simulink model "Pend_Model"  (Simulink 8.1)
settings: Solver=ode45  StartTime=0.0  StopTime=10.0  RelTol=1e-3
values from neighbouring files (symbols this model uses):
  b = 0.1    [pendulum.m]    (also in pid.m; pid_control.m)
  g = 9.8    [FastAHCCartPole.m]    (also in pendulum.m; pid.m; pid_control.m)
  l = 0.3    [pendulum.m]    (also in pid.m; pid_control.m)
  m = 0.2    [pendulum.m]    (also in pid.m; pid_control.m)
  M = 0.5    [pendulum.m]    (also in pid.m; pid_control.m)
  T = feedback(P_pend,C)    [pendulum.m]    (also in pid.m; pid_control.m)
settings Model: Creator=david78k  LastModifiedBy=david78k
settings DataIOCC: SignalLoggingSaveFormat=Dataset
settings OptimizationCC: ExpressionDepthLimit=128
settings DebuggingCC: FcnCallInpInsideContextMsg=EnableAllAsError
settings GRTTargetCC: CombineOutputUpdateFcns=on  GRTInterface=off

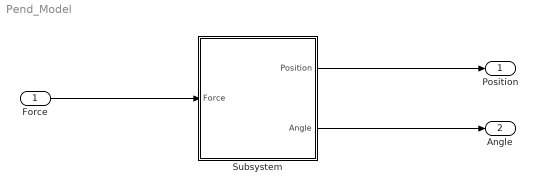
== system Pend_Model ==
  Force : Inport
  Subsystem : Subsystem
  Position : Outport
  Angle : Outport  Port=2
  wires:
  Force/1 -> Subsystem/1(Force)
  Subsystem/1(Position) -> Position/1
  Subsystem/2(Angle) -> Angle/1

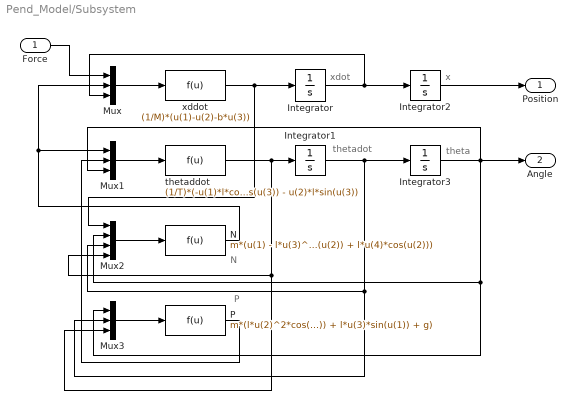
== system Pend_Model/Subsystem ==
  note: P
  note: N
  note: theta
  note: x
  note: thetadot
  note: xdot
  Force : Inport
  Integrator : Integrator  ContinuousStateAttributes='xdot'
  Integrator1 : Integrator  ContinuousStateAttributes='thetadot'
  Integrator2 : Integrator  ContinuousStateAttributes='x'
  Integrator3 : Integrator  InitialCondition=pi  ContinuousStateAttributes='theta'
  Mux : Mux  Inputs=3
  Mux1 : Mux  Inputs=3
  Mux2 : Mux
  Mux3 : Mux  Inputs=3
  N : Fcn  Expr=m*(u(1) - l*u(3)^2*sin(u(2)) + l*u(4)*cos(u(2)))
  P : Fcn  Expr=m*(l*u(2)^2*cos(u(1)) + l*u(3)*sin(u(1)) + g)
  thetaddot : Fcn  Expr=(1/T)*(-u(1)*l*cos(u(3)) - u(2)*l*sin(u(3))
  xddot : Fcn  Expr=(1/M)*(u(1)-u(2)-b*u(3))
  Position : Outport
  Angle : Outport  Port=2
  wires:
  xddot/1 -> Mux2/1, Integrator/1
  Mux1/1 -> thetaddot/1
  Integrator2/1 -> Position/1
  Integrator3/1 -> Angle/1, Mux3/1, Mux2/2, Mux1/3
  thetaddot/1 -> Mux3/3, Mux2/4, Integrator1/1
  Mux3/1 -> P/1
  Force/1 -> Mux/1
  Mux/1 -> xddot/1
  P/1 -> Mux1/2
  Integrator1/1 -> Mux3/2, Mux2/3, Integrator3/1
  Mux2/1 -> N/1
  N/1 -> Mux/2, Mux1/1
  Integrator/1 -> Integrator2/1, Mux/3
